simulink model "tp_thyr_rect_pm"  (R2024b)
settings: Solver=ode1be  StartTime=0.0  StopTime=simlength  FixedStep=tc  MaxStep=tc
undefined symbols (not defined in the file): CSF_11, CSF_13, CSF_5, CSF_7, Idc_traction_normalization_factor, ki_u_ctrl, kp_u_ctrl, LFu_dc, LSF_11, LSF_13, LSF_5, LSF_7, magnitude, n10, omega_grid_emulator_nom, pll_i1, pll_p, RLFu_dc, tc, Tcontrol_rect, ts, ts_ctrl_rect, ugrid_factor, Vdc_traction_normalization_factor, Vgrid_phase_normalization_factor, vn_eta_pu, vn_xi_pu, vp_xi_pu, w_grid
libraries: fl_lib x348, nesl_utility x85, ee_lib x28, single_phase_transformer_lib x6, cstblocks x3, spsEdgeDetectorLib x2
(part 1 of 8)
settings Model: SimulationMode=accelerator  Creator=dbagn  LastModifiedBy=ltnbda
settings SolverCC: NumberNewtonIterations=3  ZeroCrossControl=DisableAll  AlgebraicLoopSolver=TrustRegion  SolverResetMethod=Robust
settings DataIOCC: SaveOutput=off  SignalLogging=off  DSMLogging=off  SaveTime=off  ReturnWorkspaceOutputs=off
settings OptimizationCC: ReuseModelBlockBuffer=off  SimCompilerOptimization=on
settings DebuggingCC: UnconnectedInputMsg=warning  UnconnectedOutputMsg=warning  UnconnectedLineMsg=warning
settings ModelReferenceCC: EnableRefExpFcnMdlSchedulingChecks=on
settings SFSimCC: CustomCodeUndefinedFunction=ThrowError
settings SFSimCC: SimCustomHeaderCode=|
  | #include "math_f.h"
  | #include "mavgflt.h"
  | #include "mavgflt_simulink.h"
  | #include "bemf_obsv.h"
  | #include "bemf_obsv_simulink.h"
  | #include "bemf_obsv_load_est.h"
  | #include "bemf_obsv_load_est_simulink.h"
  | #include "dqvector_pi.h"
  | #include "dqvector_pi_simulink.h"
  | #include "sv_pwm_simulink.h"
  | #include "sv_pwm.h"
  | #include "twelve_pulse_rect.h"
  | #include "first_harmonic_tracker.h"
  | #include "first_harmonic_tracker_simulink.h"
  | #include "dqpll_thyr.h"
  | #include "dqpll_thyr_simulink.h"
  | #include "dqpll_grid.h"
  | #include "dqpll_grid_simulink.h"
  | #include "six_pulse_rect.h"
settings SFSimCC: SimUserSources=|
  | "mavgflt_simulink.c"
  | "mavgflt.c"
  | "bemf_obsv_simulink.c"
  | "bemf_obsv.c"
  | "bemf_obsv_load_est_simulink.c"
  | "bemf_obsv_load_est.c"
  | "dqvector_pi.c"
  | "dqvector_pi_simulink.c"
  | "sv_pwm_simulink.c"
  | "sv_pwm.c"
  | "twelve_pulse_rect.c"
  | "first_harmonic_tracker_simulink.c"
  | "first_harmonic_tracker.c"
  | "dqpll_thyr_simulink.c"
  | "dqpll_thyr.c"
  | "dqpll_grid_simulink.c"
  | "dqpll_grid.c"
  | "six_pulse_rect.c"
settings SFSimCC: SimUserIncludeDirs=|
  | include
  | src
settings RTWCC: GPUComputeCapability=3.5  DLArmComputeVersion=19.05

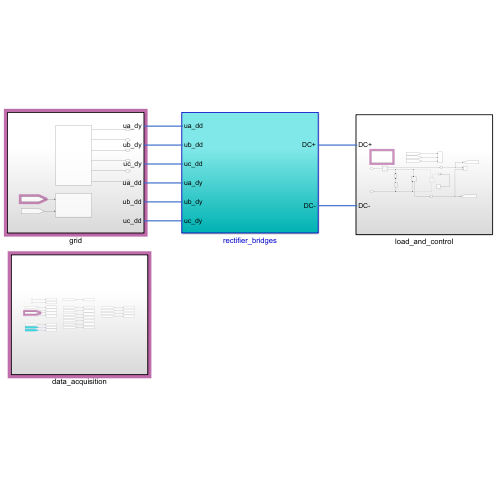
[thumbnail: Simulink's stored preview of the top-level diagram]
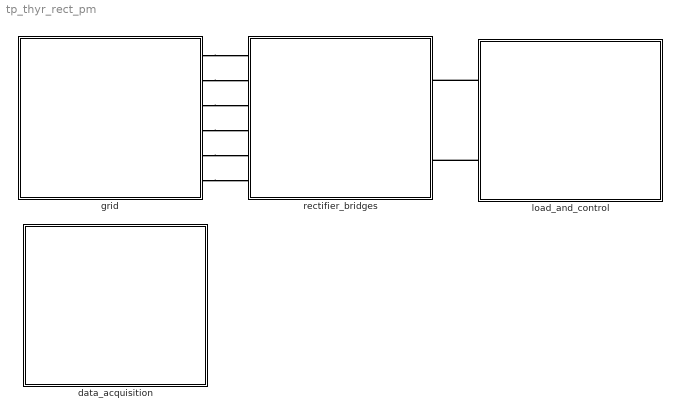
== system tp_thyr_rect_pm ==
  data_acquisition : Subsystem
  grid : Subsystem
  load_and_control : Subsystem
  rectifier_bridges : Subsystem
  connections:
  load_and_control/LConn1 -- rectifier_bridges/RConn1
  load_and_control/LConn2 -- rectifier_bridges/RConn2
  grid/RConn1 -- rectifier_bridges/LConn1
  grid/RConn2 -- rectifier_bridges/LConn2
  grid/RConn3 -- rectifier_bridges/LConn3
  grid/RConn4 -- rectifier_bridges/LConn4
  grid/RConn5 -- rectifier_bridges/LConn5
  grid/RConn6 -- rectifier_bridges/LConn6

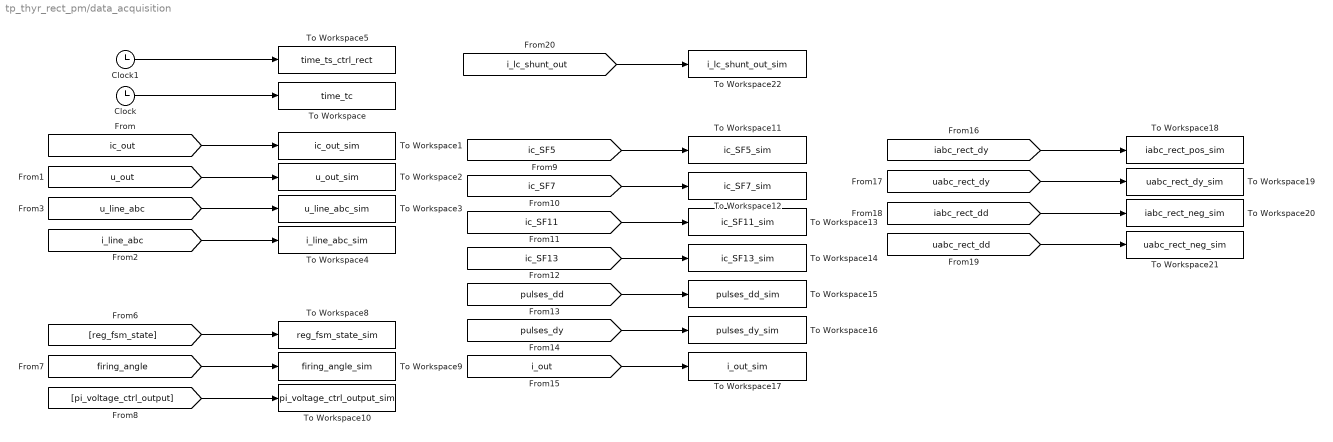
== system tp_thyr_rect_pm/data_acquisition ==
  Clock : Clock
  Clock1 : Clock
  To Workspace : ToWorkspace  VariableName=time_tc  SaveFormat=Timeseries  SampleTime=tc
      settings: MaxDataPoints=Nc
  To Workspace1 : ToWorkspace  VariableName=ic_out_sim  SaveFormat=Timeseries  SampleTime=tc
      settings: MaxDataPoints=Nc
  To Workspace10 : ToWorkspace  VariableName=pi_voltage_ctrl_output_sim  SaveFormat=Timeseries  SampleTime=ts_ctrl_rect
      settings: MaxDataPoints=Ns_ctrl_rect
  To Workspace11 : ToWorkspace  VariableName=ic_SF5_sim  SaveFormat=Timeseries  SampleTime=tc
      settings: MaxDataPoints=Nc
  To Workspace12 : ToWorkspace  VariableName=ic_SF7_sim  SaveFormat=Timeseries  SampleTime=tc
      settings: MaxDataPoints=Nc
  To Workspace13 : ToWorkspace  VariableName=ic_SF11_sim  SaveFormat=Timeseries  SampleTime=tc
      settings: MaxDataPoints=Nc
  To Workspace14 : ToWorkspace  VariableName=ic_SF13_sim  SaveFormat=Timeseries  SampleTime=tc
      settings: MaxDataPoints=Nc
  To Workspace15 : ToWorkspace  VariableName=pulses_dd_sim  SaveFormat=Timeseries  SampleTime=tc
      settings: MaxDataPoints=Nc
  To Workspace16 : ToWorkspace  VariableName=pulses_dy_sim  SaveFormat=Timeseries  SampleTime=tc
      settings: MaxDataPoints=Nc
  To Workspace17 : ToWorkspace  VariableName=i_out_sim  SaveFormat=Timeseries  SampleTime=tc
      settings: MaxDataPoints=Nc
  To Workspace18 : ToWorkspace  VariableName=iabc_rect_pos_sim  SaveFormat=Timeseries  SampleTime=tc
      settings: MaxDataPoints=Nc
  To Workspace19 : ToWorkspace  VariableName=uabc_rect_dy_sim  SaveFormat=Timeseries  SampleTime=tc
      settings: MaxDataPoints=Nc
  To Workspace2 : ToWorkspace  VariableName=u_out_sim  SaveFormat=Timeseries  SampleTime=tc
      settings: MaxDataPoints=Nc
  To Workspace20 : ToWorkspace  VariableName=iabc_rect_neg_sim  SaveFormat=Timeseries  SampleTime=tc
      settings: MaxDataPoints=Nc
  To Workspace21 : ToWorkspace  VariableName=uabc_rect_neg_sim  SaveFormat=Timeseries  SampleTime=tc
      settings: MaxDataPoints=Nc
  To Workspace22 : ToWorkspace  VariableName=i_lc_shunt_out_sim  SaveFormat=Timeseries  SampleTime=tc
      settings: MaxDataPoints=Nc
  To Workspace3 : ToWorkspace  VariableName=u_line_abc_sim  SaveFormat=Timeseries  SampleTime=tc
      settings: MaxDataPoints=Nc
  To Workspace4 : ToWorkspace  VariableName=i_line_abc_sim  SaveFormat=Timeseries  SampleTime=tc
      settings: MaxDataPoints=Nc
  To Workspace5 : ToWorkspace  VariableName=time_ts_ctrl_rect  SaveFormat=Timeseries  SampleTime=tc
      settings: MaxDataPoints=Nc
  To Workspace8 : ToWorkspace  VariableName=reg_fsm_state_sim  SaveFormat=Timeseries  SampleTime=ts_ctrl_rect
      settings: MaxDataPoints=Ns_ctrl_rect
  To Workspace9 : ToWorkspace  VariableName=firing_angle_sim  SaveFormat=Timeseries  SampleTime=ts_ctrl_rect
      settings: MaxDataPoints=Ns_ctrl_rect
  wires:
  [ic_out] -> To Workspace1/1
  Clock/1 -> To Workspace/1
  [u_line_abc] -> To Workspace3/1
  [i_line_abc] -> To Workspace4/1
  [u_out] -> To Workspace2/1
  Clock1/1 -> To Workspace5/1
  [reg_fsm_state] -> To Workspace8/1
  [firing_angle] -> To Workspace9/1
  [pi_voltage_ctrl_output] -> To Workspace10/1
  [ic_SF5] -> To Workspace11/1
  [ic_SF7] -> To Workspace12/1
  [ic_SF11] -> To Workspace13/1
  [ic_SF13] -> To Workspace14/1
  [pulses_dd] -> To Workspace15/1
  [pulses_dy] -> To Workspace16/1
  [i_out] -> To Workspace17/1
  [iabc_rect_dy] -> To Workspace18/1
  [uabc_rect_dy] -> To Workspace19/1
  [uabc_rect_dd] -> To Workspace21/1
  [iabc_rect_dd] -> To Workspace20/1
  [i_lc_shunt_out] -> To Workspace22/1

== system tp_thyr_rect_pm/grid ==
  grid_emulator : Subsystem
  instantaneus_power : Subsystem
  ua_dy : PMIOPort  Side=Right
  ub_dy : PMIOPort  Port=2  Side=Right
  uc_dy : PMIOPort  Port=3  Side=Right
  ua_dd : PMIOPort  Port=4  Side=Right
  ub_dd : PMIOPort  Port=5  Side=Right
  uc_dd : PMIOPort  Port=6  Side=Right
  wires:
  [u_line_abc] -> instantaneus_power/1(Vline)
  [i_line_abc] -> instantaneus_power/2(Iline)
  connections:
  ua_dy/RConn1 -- grid_emulator/RConn4
  ub_dy/RConn1 -- grid_emulator/RConn5
  uc_dy/RConn1 -- grid_emulator/RConn6
  ua_dd/RConn1 -- grid_emulator/RConn1
  ub_dd/RConn1 -- grid_emulator/RConn2
  uc_dd/RConn1 -- grid_emulator/RConn3

== system tp_thyr_rect_pm/load_and_control ==
  Controlled Current Source : fl_lib/Electrical/Electrical Sources/Controlled Current Source  Commented=on
  Current Sensor : fl_lib/Electrical/Electrical Sensors/Current Sensor
  Inductor : fl_lib/Electrical/Electrical Elements/Inductor  l=20e-3 H  r=0 Ohm  g=1e-9 1/Ohm  i_specify=off  i_priority=None  i=0 A  i_nominal_specify=off  i_nominal_value=1  i_nominal_unit=A  v_specify=off  v_priority=None  v=0 V  v_nominal_specify=off  v_nominal_value=1  v_nominal_unit=V  i_L_specify=off  i_L_priority=High  i_L=0 A  i_L_nominal_specify=off  i_L_nominal_value=1  i_L_nominal_unit=A
  PS-Simulink Converter : nesl_utility/PS-Simulink Converter  PhysicalDomain=network_engine_domain  SubClassName=ps_output  LeftPortType=input  RightPortType=output  PseudoPeriodic=off  Frequencies=[]  VectorFormat=1-D array  Unit=A  AffineConversion=off
  PS-Simulink Converter1 : nesl_utility/PS-Simulink Converter  PhysicalDomain=network_engine_domain  SubClassName=ps_output  LeftPortType=input  RightPortType=output  PseudoPeriodic=off  Frequencies=[]  VectorFormat=1-D array  Unit=V  AffineConversion=on
  Resistor : fl_lib/Electrical/Electrical Elements/Resistor  R=1 Ohm  i_specify=off  i_priority=None  i=0 A  i_nominal_specify=off  i_nominal_value=1  i_nominal_unit=A  v_specify=off  v_priority=None  v=0 V  v_nominal_specify=off  v_nominal_value=1  v_nominal_unit=V
  Simulink-PS Converter : nesl_utility/Simulink-PS Converter  PhysicalDomain=network_engine_domain  SubClassName=ps_input  LeftPortType=input  RightPortType=output  PseudoPeriodic=off  Frequencies=[]  NoiseDistribution=none  NoiseParameters=[]  Unit=1  AffineConversion=off  FilteringAndDerivatives=provide  SimscapeFilterOrder=1  InputFilterTimeConstant=0.001  UdotUserProvided=0
  Sine Wave : Sin  Amplitude=Idc_traction_normalization_factor/2  Bias=Idc_traction_normalization_factor/2  Frequency=pi/2  SampleTime=0
  Voltage Sensor : fl_lib/Electrical/Electrical Sensors/Voltage Sensor
  controller : Subsystem
  iu_out : Scope  NumInputPorts=2
  ui_Cout : Scope  NumInputPorts=3
  DC+ : PMIOPort  Side=Left
  DC- : PMIOPort  Port=2  Side=Left
  tag scope: i_out=global, u_out=global
  wires:
  PS-Simulink Converter/1 -> [i_out], iu_out/1  "i_out"
  PS-Simulink Converter1/1 -> [u_out], iu_out/2  "u_out"
  Sine Wave/1 -> Simulink-PS Converter/1
  [u_out] -> ui_Cout/2  "u_out"
  [ic_out] -> ui_Cout/1  "ic_out"
  [i_lc_shunt_out] -> ui_Cout/3  "i_lc_shunt_out"
  connections:
  Voltage Sensor/RConn1 -- PS-Simulink Converter1/LConn1
  Simulink-PS Converter/RConn1 -- Controlled Current Source/RConn1
  Voltage Sensor/LConn1 -- Controlled Current Source/RConn2 -- Resistor/LConn1 -- Current Sensor/RConn2
  PS-Simulink Converter/LConn1 -- Current Sensor/RConn1
  DC-/RConn1 -- Inductor/RConn1 -- Controlled Current Source/LConn1 -- Voltage Sensor/RConn2
  Inductor/LConn1 -- Resistor/RConn1
  Current Sensor/LConn1 -- DC+/RConn1

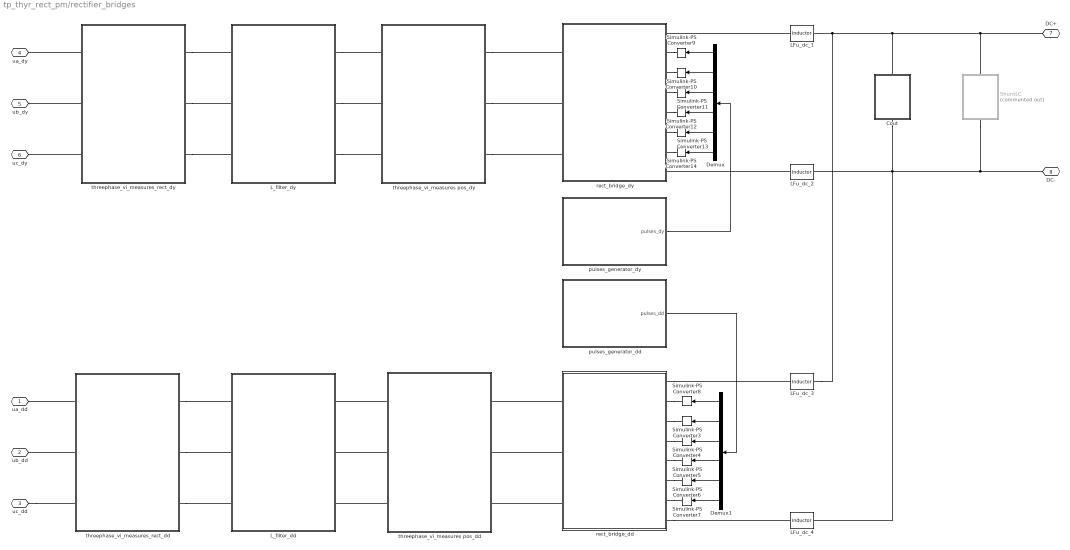
== system tp_thyr_rect_pm/rectifier_bridges ==
  Cout : Subsystem
  Demux : Demux  Outputs=6
  Demux1 : Demux  Outputs=6
  LFu_dc_{1..4} (4 alike) : fl_lib/Electrical/Electrical Elements/Inductor  l=LFu_dc/2 H  r=RLFu_dc/2 Ohm  g=1e-9 1/Ohm  i_specify=off  i_priority=None  i=0 A  i_nominal_specify=off  i_nominal_value=1  i_nominal_unit=A  v_specify=off  v_priority=None  v=0 V  v_nominal_specify=off  v_nominal_value=1  v_nominal_unit=V  i_L_specify=off  i_L_priority=High  i_L=0 A  i_L_nominal_specify=off  i_L_nominal_value=1  i_L_nominal_unit=A
  L_filter_dd : Subsystem
  L_filter_dy : Subsystem
  ShuntLC : Subsystem  Commented=on
  Simulink-PS Converter{3,5..10,12..14} (10 alike) : nesl_utility/Simulink-PS Converter  PhysicalDomain=network_engine_domain  SubClassName=ps_input  LeftPortType=input  RightPortType=output  PseudoPeriodic=off  Frequencies=[]  NoiseDistribution=none  NoiseParameters=[]  Unit=V  AffineConversion=on  FilteringAndDerivatives=provide  SimscapeFilterOrder=1  InputFilterTimeConstant=0.001  UdotUserProvided=0
  Simulink-PS Converter11 : nesl_utility/Simulink-PS Converter  PhysicalDomain=network_engine_domain  SubClassName=ps_input  LeftPortType=input  RightPortType=output  PseudoPeriodic=off  Frequencies=[]  NoiseDistribution=none  NoiseParameters=[]  Unit=V  AffineConversion=off  FilteringAndDerivatives=provide  SimscapeFilterOrder=1  InputFilterTimeConstant=0.001  UdotUserProvided=0
  Simulink-PS Converter4 : nesl_utility/Simulink-PS Converter  PhysicalDomain=network_engine_domain  SubClassName=ps_input  LeftPortType=input  RightPortType=output  PseudoPeriodic=off  Frequencies=[]  NoiseDistribution=none  NoiseParameters=[]  Unit=V  AffineConversion=off  FilteringAndDerivatives=provide  SimscapeFilterOrder=1  InputFilterTimeConstant=0.001  UdotUserProvided=0
  pulses_generator_dd : Subsystem
  pulses_generator_dy : Subsystem
  rect_bridge_dd : Subsystem
  rect_bridge_dy : Subsystem
  threephase_vi_measures pos_dd : Subsystem
  threephase_vi_measures pos_dy : Subsystem
  threephase_vi_measures_rect_dd : Subsystem
  threephase_vi_measures_rect_dy : Subsystem
  ua_dd : PMIOPort  Side=Left
  ub_dd : PMIOPort  Port=2  Side=Left
  uc_dd : PMIOPort  Port=3  Side=Left
  ua_dy : PMIOPort  Port=4  Side=Left
  ub_dy : PMIOPort  Port=5  Side=Left
  uc_dy : PMIOPort  Port=6  Side=Left
  DC+ : PMIOPort  Port=7  Side=Right
  DC- : PMIOPort  Port=8  Side=Right
  wires:
  Demux1/1 -> Simulink-PS Converter8/1
  Demux/6 -> Simulink-PS Converter14/1
  Demux1/4 -> Simulink-PS Converter5/1
  Demux1/6 -> Simulink-PS Converter7/1
  Demux1/3 -> Simulink-PS Converter4/1
  Demux/4 -> Simulink-PS Converter12/1
  Demux1/2 -> Simulink-PS Converter3/1
  Demux/1 -> Simulink-PS Converter9/1
  Demux/2 -> Simulink-PS Converter10/1
  Demux/3 -> Simulink-PS Converter11/1
  Demux1/5 -> Simulink-PS Converter6/1
  Demux/5 -> Simulink-PS Converter13/1
  pulses_generator_dd/1(pulses_dd) -> Demux1/1
  pulses_generator_dy/1(pulses_dy) -> Demux/1
  connections:
  rect_bridge_dy/LConn3 -- Simulink-PS Converter10/RConn1
  rect_bridge_dd/LConn6 -- Simulink-PS Converter6/RConn1
  rect_bridge_dd/LConn5 -- Simulink-PS Converter5/RConn1
  rect_bridge_dy/LConn5 -- Simulink-PS Converter12/RConn1
  rect_bridge_dd/LConn2 -- Simulink-PS Converter8/RConn1
  rect_bridge_dy/LConn2 -- Simulink-PS Converter9/RConn1
  rect_bridge_dd/LConn3 -- Simulink-PS Converter3/RConn1
  rect_bridge_dy/LConn4 -- Simulink-PS Converter11/RConn1
  rect_bridge_dd/LConn7 -- Simulink-PS Converter7/RConn1
  rect_bridge_dy/LConn6 -- Simulink-PS Converter13/RConn1
  rect_bridge_dy/LConn7 -- Simulink-PS Converter14/RConn1
  rect_bridge_dd/LConn4 -- Simulink-PS Converter4/RConn1
  L_filter_dy/LConn2 -- threephase_vi_measures pos_dy/LConn2
  L_filter_dy/LConn1 -- threephase_vi_measures pos_dy/LConn1
  L_filter_dy/LConn3 -- threephase_vi_measures pos_dy/LConn3
  threephase_vi_measures pos_dy/RConn1 -- rect_bridge_dy/RConn1
  threephase_vi_measures pos_dy/RConn2 -- rect_bridge_dy/RConn2
  threephase_vi_measures pos_dy/RConn3 -- rect_bridge_dy/RConn3
  rect_bridge_dd/RConn1 -- threephase_vi_measures pos_dd/RConn1
  rect_bridge_dd/RConn2 -- threephase_vi_measures pos_dd/RConn2
  rect_bridge_dd/RConn3 -- threephase_vi_measures pos_dd/RConn3
  LFu_dc_4/RConn1 -- LFu_dc_2/RConn1 -- Cout/RConn1 -- ShuntLC/RConn1 -- DC-/RConn1
  LFu_dc_1/RConn1 -- LFu_dc_3/RConn1 -- Cout/LConn1 -- ShuntLC/LConn1 -- DC+/RConn1
  LFu_dc_1/LConn1 -- rect_bridge_dy/LConn1
  LFu_dc_2/LConn1 -- rect_bridge_dy/LConn8
  rect_bridge_dd/LConn1 -- LFu_dc_3/LConn1
  rect_bridge_dd/LConn8 -- LFu_dc_4/LConn1
  threephase_vi_measures pos_dd/LConn3 -- L_filter_dd/LConn3
  threephase_vi_measures pos_dd/LConn1 -- L_filter_dd/LConn1
  threephase_vi_measures pos_dd/LConn2 -- L_filter_dd/LConn2
  threephase_vi_measures_rect_dy/RConn3 -- L_filter_dy/RConn3
  threephase_vi_measures_rect_dy/RConn2 -- L_filter_dy/RConn2
  threephase_vi_measures_rect_dy/RConn1 -- L_filter_dy/RConn1
  threephase_vi_measures_rect_dy/LConn1 -- ua_dy/RConn1
  threephase_vi_measures_rect_dy/LConn2 -- ub_dy/RConn1
  threephase_vi_measures_rect_dy/LConn3 -- uc_dy/RConn1
  threephase_vi_measures_rect_dd/LConn1 -- ua_dd/RConn1
  threephase_vi_measures_rect_dd/RConn1 -- L_filter_dd/RConn1
  threephase_vi_measures_rect_dd/RConn2 -- L_filter_dd/RConn2
  threephase_vi_measures_rect_dd/RConn3 -- L_filter_dd/RConn3
  uc_dd/RConn1 -- threephase_vi_measures_rect_dd/LConn3
  threephase_vi_measures_rect_dd/LConn2 -- ub_dd/RConn1

== system tp_thyr_rect_pm/grid/grid_emulator ==
  3ph_Dyg : Subsystem  Commented=on
  3ph_Yyg : Subsystem  Commented=on
  Controlled Voltage Source : fl_lib/Electrical/Electrical Sources/Controlled Voltage Source
  Controlled Voltage Source1 : fl_lib/Electrical/Electrical Sources/Controlled Voltage Source
  Controlled Voltage Source2 : fl_lib/Electrical/Electrical Sources/Controlled Voltage Source
  Electrical Reference : fl_lib/Electrical/Electrical Elements/Electrical Reference
  Phase Splitter : ee_lib/Connectors & References/Phase Splitter
  Phase Splitter1 : ee_lib/Connectors & References/Phase Splitter
  Phase Splitter2 : ee_lib/Connectors & References/Phase Splitter
  Simulink-PS Converter : nesl_utility/Simulink-PS Converter  PhysicalDomain=network_engine_domain  SubClassName=ps_input  LeftPortType=input  RightPortType=output  PseudoPeriodic=off  Frequencies=[]  NoiseDistribution=none  NoiseParameters=[]  Unit=V  AffineConversion=on  FilteringAndDerivatives=provide  SimscapeFilterOrder=1  InputFilterTimeConstant=0.001  UdotUserProvided=0
  Simulink-PS Converter1 : nesl_utility/Simulink-PS Converter  PhysicalDomain=network_engine_domain  SubClassName=ps_input  LeftPortType=input  RightPortType=output  PseudoPeriodic=off  Frequencies=[]  NoiseDistribution=none  NoiseParameters=[]  Unit=V  AffineConversion=on  FilteringAndDerivatives=provide  SimscapeFilterOrder=1  InputFilterTimeConstant=0.001  UdotUserProvided=0
  Simulink-PS Converter2 : nesl_utility/Simulink-PS Converter  PhysicalDomain=network_engine_domain  SubClassName=ps_input  LeftPortType=input  RightPortType=output  PseudoPeriodic=off  Frequencies=[]  NoiseDistribution=none  NoiseParameters=[]  Unit=V  AffineConversion=on  FilteringAndDerivatives=provide  SimscapeFilterOrder=1  InputFilterTimeConstant=0.001  UdotUserProvided=0
  Solver Configuration : nesl_utility/Solver Configuration  PhysicalDomain=network_engine_domain  SubClassName=solver  LeftPortType=input  RightPortType=generic  Tones=[]  Harmonics=[]  SimulateNoise=off  Profile=off  UseLocalSampling=off  EnableSwitchedLinearOptims=on  FrequencyDomain=off  UseCCode=off  RelTol=0.001  AbsTol=0.001  MinStep=1e-09  ToWorkspace=off  RevertToSquareIcSolve=off  NumHomotopyIterations=100  PhasorMode=off  PhasorModeNumHarmonics=1  ConsistencySolver=NEWTON_FTOL  IndexReductionMethod=DerivativeReplacement  DoDC=off  ResidualTolerance=1e-09  ConsistencyTolSource=GLOBAL  ConsistencyAbsTol=0.001  ConsistencyRelTol=0.001  ConsistencyTolFactor=0.001  UseLocalSolver=on  LocalSolverChoice=NE_BACKWARD_EULER_ADVANCER  ResolveIndetEquations=on  FunctionEvalNumThread=1  LocalSolverSampleTime=tc  DoFixedCost=on  MaxNonlinIter=3  MaxModeIter=2  ComputeImpulses=off  ImpulseIterations=2  LinearAlgebra=auto  LinearAlgebraNumThread=0  EquationFormulation=NE_TIME_EF  DelaysMemoryBudget=1024  AutomaticFiltering=on  FilteringTimeConstant=0.001  PartitionStorageMethod=AS_NEEDED  PartitionMemoryBudget=1024  PartitionMethod=ROBUST  MultibodyUseLocalSolver=off  MultibodyLocalSolverChoice=ODE1  MultibodyLocalSolverSampleTime=0.001
  Three-Winding Transformer (Three-Phase) : ee_lib/Passive/Transformers/Three-Winding Transformer (Three-Phase)  SRated=1.6e6 A*V  FRated=50 Hz  Winding1Connection=ee.enum.windingconnection.delta11  VRated1=400 V  Winding2Connection=ee.enum.windingconnection.delta1  VRated2=400 V  Winding3Connection=ee.enum.windingconnection.Y  VRated3=400 V  CoreType=ee.enum.coretype.threelimb  pu_Rw1=0.02  pu_Rw2=0.02  pu_Rw3=0.02  leakage_reactance_option=ee.enum.transformer_leakage.include  pu_Xl1=0.05  pu_Xl2=0.05  pu_Xl3=0.05  magnetizing_resistance_option=ee.enum.transformer_magnetizingResistance.include  pu_Rm=500  magnetizing_reactance_option=ee.enum.transformer_magnetizingReactance.include  saturation_option=ee.enum.transformer_saturation.exclude  pu_Xm=500  current_data=[0, .002, 1, 2]  magnetic_flux_data=[0, 1.2, 1.5, 1.51]  pu_X0=0.5  i1_specify=off  i1_priority=None  i1=[0, 0, 0] A  i1_nominal_specify=off  i1_nominal_value=1  i1_nominal_unit=A  i2_specify=off  i2_priority=None  i2=[0, 0, 0] A  i2_nominal_specify=off  i2_nominal_value=1  i2_nominal_unit=A  i3_specify=off  i3_priority=None  i3=[0, 0, 0] A  i3_nominal_specify=off  i3_nominal_value=1  i3_nominal_unit=A  phi_specify=off  phi_priority=None  phi=[0, 0, 0]  phi_nominal_specify=off  phi_nominal_value=1  phi_nominal_unit=1  power_dissipated_specify=off  power_dissipated_priority=None  power_dissipated=0 W  power_dissipated_nominal_specify=off  power_dissipated_nominal_value=1  power_dissipated_nominal_unit=W
      settings: InternalSimscapePortConfiguration="{\"Bottom\":[],\"Left\":[{\"id\":\"N1\",\"label\":\"~1\",\"type\":\"foundation.electrical.three_phase\"}],\"Right\":[{\"id\":\"N2\",\"label\":\"~2\",\"type\":\"foundation.electrical.three_phase\"},{\"id\":\"N3\",\"label\":\"~3\",\"type\":\"foundation.electrical.three_phase\"}],\"Top\":[]}"
  grid_emulator : Subsystem
  threephase_vi_measures : Subsystem
  ua_dd : PMIOPort  Side=Right
  ub_dd : PMIOPort  Port=2  Side=Right
  uc_dd : PMIOPort  Port=3  Side=Right
  ua_dy : PMIOPort  Port=4  Side=Right
  ub_dy : PMIOPort  Port=5  Side=Right
  uc_dy : PMIOPort  Port=6  Side=Right
  wires:
  grid_emulator/2(Vmb) -> Simulink-PS Converter1/1
  grid_emulator/3(Vmc) -> Simulink-PS Converter2/1
  grid_emulator/1(Vma) -> Simulink-PS Converter/1
  connections:
  Simulink-PS Converter/RConn1 -- Controlled Voltage Source/RConn1
  Simulink-PS Converter1/RConn1 -- Controlled Voltage Source1/RConn1
  Simulink-PS Converter2/RConn1 -- Controlled Voltage Source2/RConn1
  Electrical Reference/LConn1 -- Solver Configuration/RConn1 -- Controlled Voltage Source/RConn2 -- Controlled Voltage Source1/RConn2 -- Controlled Voltage Source2/RConn2
  Controlled Voltage Source/LConn1 -- threephase_vi_measures/LConn1
  Controlled Voltage Source1/LConn1 -- threephase_vi_measures/LConn2
  Controlled Voltage Source2/LConn1 -- threephase_vi_measures/LConn3
  Phase Splitter/RConn3 -- threephase_vi_measures/RConn1
  threephase_vi_measures/RConn2 -- Phase Splitter/RConn2
  threephase_vi_measures/RConn3 -- Phase Splitter/RConn1
  Three-Winding Transformer (Three-Phase)/LConn1 -- Phase Splitter/LConn1
  ua_dd/RConn1 -- Phase Splitter1/RConn1
  ub_dd/RConn1 -- Phase Splitter1/RConn2
  Phase Splitter1/RConn3 -- uc_dd/RConn1
  Phase Splitter2/LConn1 -- Three-Winding Transformer (Three-Phase)/RConn2
  Phase Splitter2/RConn1 -- ua_dy/RConn1
  Phase Splitter2/RConn2 -- ub_dy/RConn1
  Phase Splitter2/RConn3 -- uc_dy/RConn1
  Three-Winding Transformer (Three-Phase)/RConn1 -- Phase Splitter1/LConn1

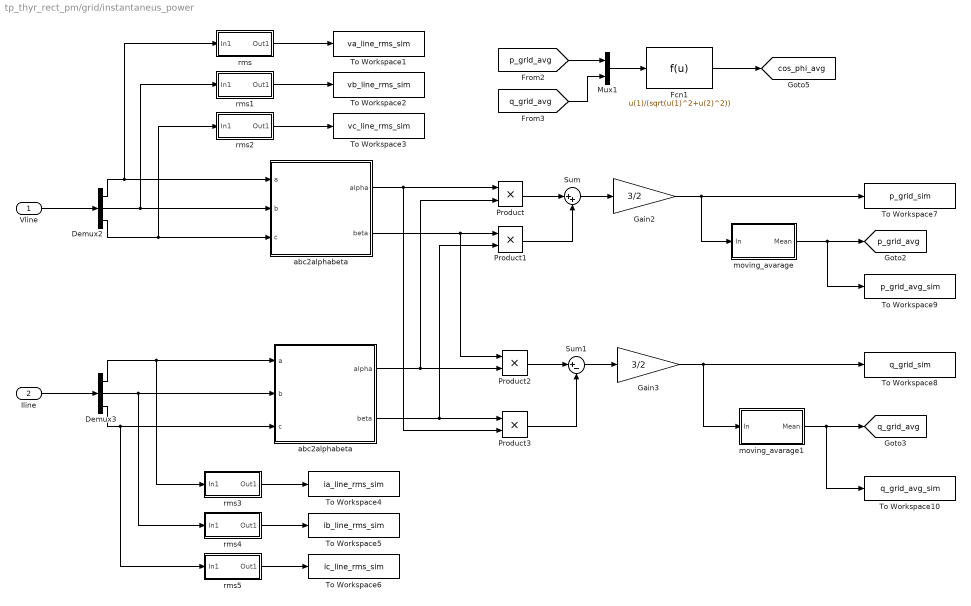
== system tp_thyr_rect_pm/grid/instantaneus_power ==
  Vline : Inport
  Iline : Inport  Port=2
  Demux2 : Demux  Outputs=3
  Demux3 : Demux  Outputs=3
  Fcn1 : Fcn  Expr=u(1)/(sqrt(u(1)^2+u(2)^2))
  Gain2 : Gain  Gain=3/2
  Gain3 : Gain  Gain=3/2
  Mux1 : Mux  Inputs=2
  Product{,1..3} (4 alike) : Product  RndMeth=Zero
  Sum : Sum  Inputs=|++
  Sum1 : Sum  Inputs=|+-
  To Workspace1 : ToWorkspace  VariableName=va_line_rms_sim  SampleTime=ts_ctrl_rect
      settings: MaxDataPoints=Ns_ctrl_rect
  To Workspace10 : ToWorkspace  VariableName=q_grid_avg_sim  SampleTime=ts_ctrl_rect
      settings: MaxDataPoints=Ns_ctrl_rect
  To Workspace2 : ToWorkspace  VariableName=vb_line_rms_sim  SampleTime=ts_ctrl_rect
      settings: MaxDataPoints=Ns_ctrl_rect
  To Workspace3 : ToWorkspace  VariableName=vc_line_rms_sim  SampleTime=ts_ctrl_rect
      settings: MaxDataPoints=Ns_ctrl_rect
  To Workspace4 : ToWorkspace  VariableName=ia_line_rms_sim  SampleTime=ts_ctrl_rect
      settings: MaxDataPoints=Ns_ctrl_rect
  To Workspace5 : ToWorkspace  VariableName=ib_line_rms_sim  SampleTime=ts_ctrl_rect
      settings: MaxDataPoints=Ns_ctrl_rect
  To Workspace6 : ToWorkspace  VariableName=ic_line_rms_sim  SampleTime=ts_ctrl_rect
      settings: MaxDataPoints=Ns_ctrl_rect
  To Workspace7 : ToWorkspace  VariableName=p_grid_sim  SampleTime=ts_ctrl_rect
      settings: MaxDataPoints=Ns_ctrl_rect
  To Workspace8 : ToWorkspace  VariableName=q_grid_sim  SampleTime=ts_ctrl_rect
      settings: MaxDataPoints=Ns_ctrl_rect
  To Workspace9 : ToWorkspace  VariableName=p_grid_avg_sim  SampleTime=ts_ctrl_rect
      settings: MaxDataPoints=Ns_ctrl_rect
  abc2alphabeta : Subsystem
  "abc2alphabeta " : Subsystem
  moving_avarage : Subsystem
  moving_avarage1 : Subsystem
  rms : Subsystem
  rms1 : Subsystem
  rms2 : Subsystem
  rms3 : Subsystem
  rms4 : Subsystem
  rms5 : Subsystem
  tag scope: cos_phi_avg=global, p_grid_avg=global, q_grid_avg=global
  wires:
  Gain3/1 -> moving_avarage1/1(In), To Workspace8/1
  Gain2/1 -> moving_avarage/1(In), To Workspace7/1
  Demux2/1 -> abc2alphabeta/1(a), rms/1(In1)
  Vline/1 -> Demux2/1
  Iline/1 -> Demux3/1
  abc2alphabeta/2("beta ") -> Product1/1, Product2/1
  "abc2alphabeta "/2("beta ") -> Product3/1, Product1/2
  abc2alphabeta/1("alpha ") -> Product/1, Product3/2
  "abc2alphabeta "/1("alpha ") -> Product2/2, Product/2
  Product/1 -> Sum/1
  Product1/1 -> Sum/2
  Product2/1 -> Sum1/1
  Product3/1 -> Sum1/2
  Sum1/1 -> Gain3/1
  Sum/1 -> Gain2/1
  Demux2/2 -> abc2alphabeta/2(b), rms1/1(In1)
  Demux2/3 -> abc2alphabeta/3(c), rms2/1(In1)
  Demux3/1 -> rms3/1(In1), "abc2alphabeta "/1(a)
  Demux3/2 -> rms4/1(In1), "abc2alphabeta "/2(b)
  Demux3/3 -> rms5/1(In1), "abc2alphabeta "/3(c)
  moving_avarage/1(Mean) -> [p_grid_avg], To Workspace9/1
  moving_avarage1/1(Mean) -> To Workspace10/1, [q_grid_avg]
  [q_grid_avg] -> Mux1/2
  Mux1/1 -> Fcn1/1
  Fcn1/1 -> [cos_phi_avg]
  [p_grid_avg] -> Mux1/1
  rms/1(Out1) -> To Workspace1/1
  rms2/1(Out1) -> To Workspace3/1
  rms1/1(Out1) -> To Workspace2/1
  rms5/1(Out1) -> To Workspace6/1
  rms4/1(Out1) -> To Workspace5/1
  rms3/1(Out1) -> To Workspace4/1

== system tp_thyr_rect_pm/load_and_control/controller ==
  Constant2 : Constant
  firing_angles : Scope
  pi_voltage_ctrl : Subsystem
  tag scope: firing_angle=global
  wires:
  [u_out] -> pi_voltage_ctrl/2(vout)
  Constant2/1 -> pi_voltage_ctrl/1(vout_ref)
  pi_voltage_ctrl/1(w) -> firing_angles/1, [firing_angle]

== system tp_thyr_rect_pm/rectifier_bridges/Cout ==
  Capacitor : fl_lib/Electrical/Electrical Elements/Capacitor  c=CFu_dc F  r=RCFu_dc Ohm  g=0 1/Ohm  i_specify=off  i_priority=None  i=0 A  i_nominal_specify=off  i_nominal_value=1  i_nominal_unit=A  v_specify=off  v_priority=None  v=0 V  v_nominal_specify=off  v_nominal_value=1  v_nominal_unit=V  vc_specify=off  vc_priority=High  vc=0 V  vc_nominal_specify=off  vc_nominal_value=1  vc_nominal_unit=V
  Current Sensor1 : fl_lib/Electrical/Electrical Sensors/Current Sensor
  PS-Simulink Converter2 : nesl_utility/PS-Simulink Converter  PhysicalDomain=network_engine_domain  SubClassName=ps_output  LeftPortType=input  RightPortType=output  PseudoPeriodic=off  Frequencies=[]  VectorFormat=1-D array  Unit=A  AffineConversion=off
  u+ : PMIOPort  Side=Left
  u- : PMIOPort  Port=2  Side=Right
  tag scope: ic_out=global
  wires:
  PS-Simulink Converter2/1 -> [ic_out]
  connections:
  Capacitor/RConn1 -- u-/RConn1
  Current Sensor1/RConn2 -- Capacitor/LConn1
  PS-Simulink Converter2/LConn1 -- Current Sensor1/RConn1
  Current Sensor1/LConn1 -- u+/RConn1

== system tp_thyr_rect_pm/rectifier_bridges/L_filter_dd ==
  Inductor : fl_lib/Electrical/Electrical Elements/Inductor  l=1e-6 H  r=0 Ohm  g=1e-9 1/Ohm  i_specify=on  i_priority=High  i=0 A  i_nominal_specify=off  i_nominal_value=1  i_nominal_unit=A  v_specify=off  v_priority=None  v=0 V  v_nominal_specify=off  v_nominal_value=1  v_nominal_unit=V  i_L_specify=off  i_L_priority=High  i_L=0 A  i_L_nominal_specify=off  i_L_nominal_value=1  i_L_nominal_unit=A
  Inductor1 : fl_lib/Electrical/Electrical Elements/Inductor  l=1e-6 H  r=0 Ohm  g=1e-9 1/Ohm  i_specify=on  i_priority=High  i=0 A  i_nominal_specify=off  i_nominal_value=1  i_nominal_unit=A  v_specify=off  v_priority=None  v=0 V  v_nominal_specify=off  v_nominal_value=1  v_nominal_unit=V  i_L_specify=off  i_L_priority=High  i_L=0 A  i_L_nominal_specify=off  i_L_nominal_value=1  i_L_nominal_unit=A
  Inductor2 : fl_lib/Electrical/Electrical Elements/Inductor  l=1e-6 H  r=0 Ohm  g=1e-9 1/Ohm  i_specify=on  i_priority=High  i=0 A  i_nominal_specify=off  i_nominal_value=1  i_nominal_unit=A  v_specify=off  v_priority=None  v=0 V  v_nominal_specify=off  v_nominal_value=1  v_nominal_unit=V  i_L_specify=off  i_L_priority=High  i_L=0 A  i_L_nominal_specify=off  i_L_nominal_value=1  i_L_nominal_unit=A
  shunt_passive_filter_11 : Subsystem  mask{CSF=CSF_11, LSF=LSF_11, RCSF=5e-3}
      mask prompts: CSF "Shunt Capacitor"; LSF "Shunt Inductor"; RCSF "Shunt Resistor"
      mask Display: disp('SPF');
  shunt_passive_filter_13 : Subsystem  mask{CSF=CSF_13, LSF=LSF_13, RCSF=5e-3}
      mask prompts: CSF "Shunt Capacitor"; LSF "Shunt Inductor"; RCSF "Shunt Resistor"
      mask Display: disp('SPF');
  shunt_passive_filter_5 : Subsystem  mask{CSF=CSF_5, LSF=LSF_5, RCSF=5e-3}
      mask prompts: CSF "Shunt Capacitor"; LSF "Shunt Inductor"; RCSF "Shunt Resistor"
      mask Display: disp('SPF');
  shunt_passive_filter_7 : Subsystem  mask{CSF=CSF_7, LSF=LSF_7, RCSF=5e-3}
      mask prompts: CSF "Shunt Capacitor"; LSF "Shunt Inductor"; RCSF "Shunt Resistor"
      mask Display: disp('SPF');
  ui_measure : Subsystem
  us_a : PMIOPort  Side=Left
  ug_a : PMIOPort  Port=2  Side=Right
  us_b : PMIOPort  Port=3  Side=Left
  ug_b : PMIOPort  Port=4  Side=Right
  us_c : PMIOPort  Port=5  Side=Left
  ug_c : PMIOPort  Port=6  Side=Right
  connections:
  ug_c/RConn1 -- ui_measure/LConn3
  ug_a/RConn1 -- ui_measure/LConn1
  ug_b/RConn1 -- ui_measure/LConn2
  Inductor2/RConn1 -- us_c/RConn1
  Inductor1/RConn1 -- us_b/RConn1
  us_a/RConn1 -- Inductor/RConn1
  shunt_passive_filter_5/RConn3 -- Inductor2/LConn1 -- shunt_passive_filter_13/RConn3 -- shunt_passive_filter_11/RConn3 -- shunt_passive_filter_7/RConn3 -- ui_measure/RConn3
  shunt_passive_filter_5/RConn2 -- Inductor1/LConn1 -- shunt_passive_filter_13/RConn2 -- shunt_passive_filter_11/RConn2 -- shunt_passive_filter_7/RConn2 -- ui_measure/RConn2
  shunt_passive_filter_5/RConn1 -- Inductor/LConn1 -- shunt_passive_filter_13/RConn1 -- shunt_passive_filter_11/RConn1 -- shunt_passive_filter_7/RConn1 -- ui_measure/RConn1

== system tp_thyr_rect_pm/rectifier_bridges/L_filter_dy ==
  Inductor : fl_lib/Electrical/Electrical Elements/Inductor  l=1e-6 H  r=0 Ohm  g=1e-9 1/Ohm  i_specify=on  i_priority=High  i=0 A  i_nominal_specify=off  i_nominal_value=1  i_nominal_unit=A  v_specify=off  v_priority=None  v=0 V  v_nominal_specify=off  v_nominal_value=1  v_nominal_unit=V  i_L_specify=off  i_L_priority=High  i_L=0 A  i_L_nominal_specify=off  i_L_nominal_value=1  i_L_nominal_unit=A
  Inductor1 : fl_lib/Electrical/Electrical Elements/Inductor  l=1e-6 H  r=0 Ohm  g=1e-9 1/Ohm  i_specify=on  i_priority=High  i=0 A  i_nominal_specify=off  i_nominal_value=1  i_nominal_unit=A  v_specify=off  v_priority=None  v=0 V  v_nominal_specify=off  v_nominal_value=1  v_nominal_unit=V  i_L_specify=off  i_L_priority=High  i_L=0 A  i_L_nominal_specify=off  i_L_nominal_value=1  i_L_nominal_unit=A
  Inductor2 : fl_lib/Electrical/Electrical Elements/Inductor  l=1e-6 H  r=0 Ohm  g=1e-9 1/Ohm  i_specify=on  i_priority=High  i=0 A  i_nominal_specify=off  i_nominal_value=1  i_nominal_unit=A  v_specify=off  v_priority=None  v=0 V  v_nominal_specify=off  v_nominal_value=1  v_nominal_unit=V  i_L_specify=off  i_L_priority=High  i_L=0 A  i_L_nominal_specify=off  i_L_nominal_value=1  i_L_nominal_unit=A
  i_SFs : Scope  NumInputPorts=4
  shunt_passive_filter_11 : Subsystem  mask{CSF=CSF_11, LSF=LSF_11, RCSF=5e-3}
      mask prompts: CSF "Shunt Capacitor"; LSF "Shunt Inductor"; RCSF "Shunt Resistor"
      mask Display: disp('SPF');
  shunt_passive_filter_13 : Subsystem  mask{CSF=CSF_13, LSF=LSF_13, RCSF=5e-3}
      mask prompts: CSF "Shunt Capacitor"; LSF "Shunt Inductor"; RCSF "Shunt Resistor"
      mask Display: disp('SPF');
  shunt_passive_filter_5 : Subsystem  mask{CSF=CSF_5, LSF=LSF_5, RCSF=5e-3}
      mask prompts: CSF "Shunt Capacitor"; LSF "Shunt Inductor"; RCSF "Shunt Resistor"
      mask Display: disp('SPF');
  shunt_passive_filter_7 : Subsystem  mask{CSF=CSF_7, LSF=LSF_7, RCSF=5e-3}
      mask prompts: CSF "Shunt Capacitor"; LSF "Shunt Inductor"; RCSF "Shunt Resistor"
      mask Display: disp('SPF');
  ui_measure : Subsystem
  us_a : PMIOPort  Side=Left
  ug_a : PMIOPort  Port=2  Side=Right
  us_b : PMIOPort  Port=3  Side=Left
  ug_b : PMIOPort  Port=4  Side=Right
  us_c : PMIOPort  Port=5  Side=Left
  ug_c : PMIOPort  Port=6  Side=Right
  wires:
  [ic_SF5] -> i_SFs/1
  [ic_SF7] -> i_SFs/2
  [ic_SF11] -> i_SFs/3
  [ic_SF13] -> i_SFs/4
  connections:
  ui_measure/RConn1 -- shunt_passive_filter_7/RConn1 -- shunt_passive_filter_11/RConn1 -- shunt_passive_filter_13/RConn1 -- Inductor/LConn1 -- shunt_passive_filter_5/RConn1
  ui_measure/RConn2 -- shunt_passive_filter_7/RConn2 -- shunt_passive_filter_11/RConn2 -- shunt_passive_filter_13/RConn2 -- Inductor1/LConn1 -- shunt_passive_filter_5/RConn2
  ui_measure/RConn3 -- shunt_passive_filter_7/RConn3 -- shunt_passive_filter_11/RConn3 -- shunt_passive_filter_13/RConn3 -- Inductor2/LConn1 -- shunt_passive_filter_5/RConn3
  us_a/RConn1 -- Inductor/RConn1
  Inductor1/RConn1 -- us_b/RConn1
  Inductor2/RConn1 -- us_c/RConn1
  ug_b/RConn1 -- ui_measure/LConn2
  ug_a/RConn1 -- ui_measure/LConn1
  ug_c/RConn1 -- ui_measure/LConn3

== system tp_thyr_rect_pm/rectifier_bridges/ShuntLC ==
  Capacitor : fl_lib/Electrical/Electrical Elements/Capacitor  c=C_shunt_dc F  r=RC_shunt_dc Ohm  g=0 1/Ohm  i_specify=off  i_priority=None  i=0 A  i_nominal_specify=off  i_nominal_value=1  i_nominal_unit=A  v_specify=off  v_priority=None  v=0 V  v_nominal_specify=off  v_nominal_value=1  v_nominal_unit=V  vc_specify=off  vc_priority=High  vc=0 V  vc_nominal_specify=off  vc_nominal_value=1  vc_nominal_unit=V
  Capacitor1 : fl_lib/Electrical/Electrical Elements/Capacitor  c=C_shunt_dc F  r=RC_shunt_dc Ohm  g=0 1/Ohm  i_specify=off  i_priority=None  i=0 A  i_nominal_specify=off  i_nominal_value=1  i_nominal_unit=A  v_specify=off  v_priority=None  v=0 V  v_nominal_specify=off  v_nominal_value=1  v_nominal_unit=V  vc_specify=off  vc_priority=High  vc=0 V  vc_nominal_specify=off  vc_nominal_value=1  vc_nominal_unit=V
  Current Sensor1 : fl_lib/Electrical/Electrical Sensors/Current Sensor
  Inductor : fl_lib/Electrical/Electrical Elements/Inductor  l=L_shunt_dc H  r=0 Ohm  g=1e-9 1/Ohm  i_specify=off  i_priority=None  i=0 A  i_nominal_specify=off  i_nominal_value=1  i_nominal_unit=A  v_specify=off  v_priority=None  v=0 V  v_nominal_specify=off  v_nominal_value=1  v_nominal_unit=V  i_L_specify=off  i_L_priority=High  i_L=0 A  i_L_nominal_specify=off  i_L_nominal_value=1  i_L_nominal_unit=A
  PS-Simulink Converter2 : nesl_utility/PS-Simulink Converter  PhysicalDomain=network_engine_domain  SubClassName=ps_output  LeftPortType=input  RightPortType=output  PseudoPeriodic=off  Frequencies=[]  VectorFormat=1-D array  Unit=A  AffineConversion=off
  u+ : PMIOPort  Side=Left
  u- : PMIOPort  Port=2  Side=Right
  tag scope: i_lc_shunt_out=global
  wires:
  PS-Simulink Converter2/1 -> [i_lc_shunt_out]
  connections:
  Current Sensor1/LConn1 -- u+/RConn1
  PS-Simulink Converter2/LConn1 -- Current Sensor1/RConn1
  Current Sensor1/RConn2 -- Capacitor1/LConn1 -- Capacitor/LConn1
  Capacitor/RConn1 -- Capacitor1/RConn1 -- Inductor/LConn1
  Inductor/RConn1 -- u-/RConn1

== system tp_thyr_rect_pm/rectifier_bridges/pulses_generator_dd ==
  C-caller ctrl : Subsystem
  Step : Step  Time=0  Before=1  After=0
  pll : Subsystem
  pulses_dd : Outport
  wires:
  [firing_angle] -> C-caller ctrl/1(alpha)
  C-caller ctrl/1(pulses_dy) -> pulses_dd/1
  Step/1 -> C-caller ctrl/3(Block)
  pll/1(grid_phase_hat) -> C-caller ctrl/2(grid_phase)

== system tp_thyr_rect_pm/rectifier_bridges/pulses_generator_dy ==
  C-caller ctrl : Subsystem
  Step : Step  Time=0  Before=1  After=0
  pll : Subsystem
  pulses_dy : Outport
  wires:
  pll/1(grid_phase_hat) -> C-caller ctrl/2(grid_phase)
  Step/1 -> C-caller ctrl/3(Block)
  C-caller ctrl/1(pulses_dy) -> pulses_dy/1
  [firing_angle] -> C-caller ctrl/1(alpha)

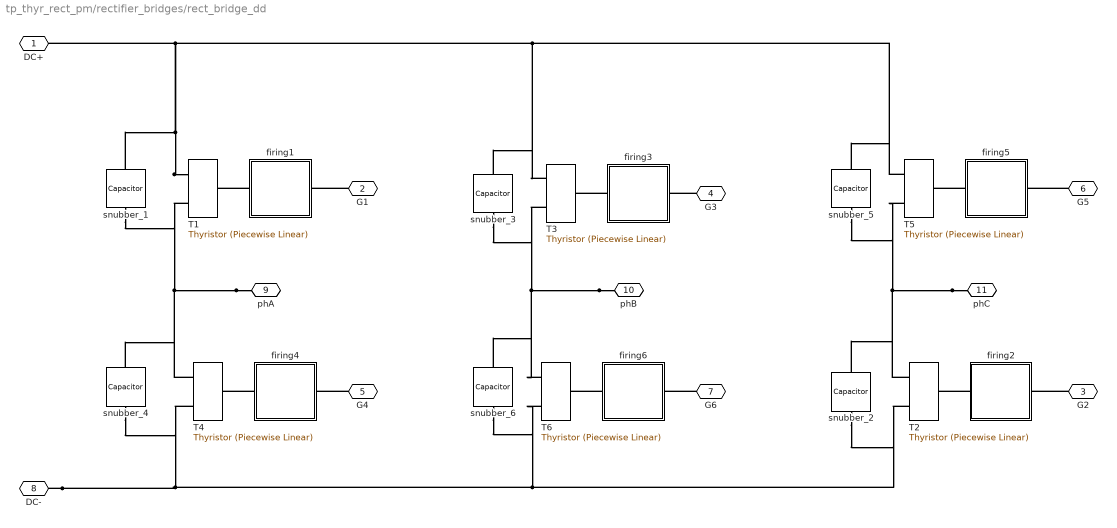
== system tp_thyr_rect_pm/rectifier_bridges/rect_bridge_dd ==
  T{1..6} (6 alike) : ee_lib/Semiconductors & Converters/Thyristor (Piecewise Linear)  port_option=ee.enum.controlport.ps  Vf=0.8 V  Ron=0.001 Ohm  Goff=1e-5 1/Ohm  Vgt=6 V  Ih=1 A  diode_param=1  diode_Vf=0.8 V  diode_Ron=0.001 Ohm  diode_Goff=1e-5 1/Ohm  diode_C=50e-9 F  diode_iRM=-235 A  diode_iF=300 A  diode_idot=-50 A/us  diode_trr_param=1  diode_trr_factor=3  diode_trr=15 us  diode_Qrr=1500 s*uA  iak_specify=off  iak_priority=None  iak=0 A  iak_nominal_specify=off  iak_nominal_value=1  iak_nominal_unit=A  vak_specify=off  vak_priority=None  vak=0 V  vak_nominal_specify=off  vak_nominal_value=1  vak_nominal_unit=V  vgk_specify=off  vgk_priority=None  vgk=0 V  vgk_nominal_specify=off  vgk_nominal_value=1  vgk_nominal_unit=V  thermal_loss_option=2  Von_data=[0, 1.1, 1.3, 1.45, 1.75, 2.25, 2.7; 0, 1, 1.15, 1.35, 1.7, 2.35, 3] V  Tj=[298.15, 398.15] K  Iout_data=[0, 10, 50, 100, 200, 400, 600] A  Eon_data=[0, .29, 1.43, 2.86, 5.71, 13.14, 22.86; 0, .57, 2.63, 5.14, 10.29, 20.57, 30.29] * 1e-3 J  Tj_loss=[298.15, 398.15] K  Iout_data_loss=[0, .1, 1, 5, 10, 20, 40, 70, 100] A  Eon_scalar=22.86e-3 J  Eoff_natural_commutation=10e-3 J  Voff=300 V  Iout_scalar=600 A  onCurrentMeasDelay=1e-4 s  diodeModelType=ee.enum.converters.diodeModelType.pwl  diodeTableType=ee.enum.diode.tableType.IfMat  diode_IfMat=[.07, .12, .19, 1.75, 4.24, 7.32, 11.2; .16, .3, .72, 2.14, 4.02, 6.35, 9.12] A  diode_VfMat=[.9, 1.15, 1.25, 1.5, 1.75, 2.17, 2.6, 2.85; .58, .68, .75, 1.1, 1.38, 1.77, 2.27, 2.7] V  diode_TjVec=[25, 125] degC  diode_VfVec=[.5, .7, .9, 1.3, 1.7, 2.1, 2.5] V  diode_IfVec=[.1, .2, .5, 1, 2, 4, 7, 10] A  diode_rec_loss_model=ee.enum.diode.reverseRecoveryModel.fixed  diode_ErecVal=0 J  diode_scaleWithIandV=true  diode_ErecMat=zeros(2, 3) J  diode_TjrecVec=[298.15, 398.15] K  diode_IfrecVec=[.1, 1, 10] A  diode_IrecVal=10 A  diode_VrecVal=10 V  diode_tFilter=1 / 1000 / 100 s  thermal_network_parameterization=ee.enum.thermalNetworkTopology.external  Rth=[.08, .5] K/W  Rth_Cauer=[.08, .1, .5] K/W  Rth_Foster=[.08, .14, .22, .16] K/W  thermal_mass_parameterization=ee.enum.thermalNetwork.timeconstant  thermal_mass=[.01, .5] J/K  thermal_mass_Cauer=[.01, .1, .5] J/K  thermal_mass_Foster=[.001, .005, .05, .5] J/K  thermal_time_constant=[.001, .2] s  thermal_time_constant_Cauer=[.001, .1, .2] s  thermal_time_constant_Foster=[7e-05, .0007, .01, .08] s  thermal_mass_initial_temperatures=[25, 25] degC  thermal_mass_initial_temperatures_Cauer=[25, 25, 25] degC  junction_thermal_mass=0.01 J/K  Tvec_initial_Foster=[25, 25, 25, 25] degC  junction_temperature_specify=off  junction_temperature_priority=None  junction_temperature=25 degC  junction_temperature_nominal_specify=off  junction_temperature_nominal_value=1  junction_temperature_nominal_unit=degC  Qj_specify=off  Qj_priority=None  Qj=0 W  Qj_nominal_specify=off  Qj_nominal_value=1  Qj_nominal_unit=W  accumulatedSwitchingLosses_specify=off  accumulatedSwitchingLosses_priority=None  accumulatedSwitchingLosses=0 J
      settings: InternalSimscapePortConfiguration="{\"Bottom\":[],\"Left\":[{\"id\":\"G\",\"label\":\"\",\"type\":\"input\"}],\"Right\":[{\"id\":\"A\",\"label\":\"\",\"type\":\"foundation.electrical.electrical\"},{\"id\":\"K\",\"label\":\"\",\"type\":\"foundation.electrical.electrical\"}],\"Top\":[]}"
  firing1 : Subsystem
  firing2 : Subsystem
  firing3 : Subsystem
  firing4 : Subsystem
  firing5 : Subsystem
  firing6 : Subsystem
  snubber_{1..6} (6 alike) : fl_lib/Electrical/Electrical Elements/Capacitor  c=Csnubber_scr F  r=Rsnubber_scr Ohm  g=0 1/Ohm  i_specify=off  i_priority=None  i=0 A  i_nominal_specify=off  i_nominal_value=1  i_nominal_unit=A  v_specify=off  v_priority=None  v=0 V  v_nominal_specify=off  v_nominal_value=1  v_nominal_unit=V  vc_specify=off  vc_priority=High  vc=0 V  vc_nominal_specify=off  vc_nominal_value=1  vc_nominal_unit=V
  DC+ : PMIOPort  Side=Left
  G1 : PMIOPort  Port=2  Side=Left
  G2 : PMIOPort  Port=3  Side=Left
  G3 : PMIOPort  Port=4  Side=Left
  G4 : PMIOPort  Port=5  Side=Left
  G5 : PMIOPort  Port=6  Side=Left
  G6 : PMIOPort  Port=7  Side=Left
  DC- : PMIOPort  Port=8  Side=Left
  phA : PMIOPort  Port=9  Side=Right
  phB : PMIOPort  Port=10  Side=Right
  phC : PMIOPort  Port=11  Side=Right
  connections:
  firing6/RConn1 -- T6/LConn1
  firing5/RConn1 -- T5/LConn1
  firing4/RConn1 -- T4/LConn1
  firing3/RConn1 -- T3/LConn1
  firing2/RConn1 -- T2/LConn1
  firing1/RConn1 -- T1/LConn1
  G6/RConn1 -- firing6/LConn1
  G5/RConn1 -- firing5/LConn1
  G4/RConn1 -- firing4/LConn1
  G3/RConn1 -- firing3/LConn1
  G2/RConn1 -- firing2/LConn1
  G1/RConn1 -- firing1/LConn1
  DC-/RConn1 -- T4/RConn1 -- snubber_4/RConn1 -- T6/RConn1 -- snubber_6/RConn1 -- snubber_2/RConn1 -- T2/RConn1
  phB/RConn1 -- T6/RConn2 -- snubber_6/LConn1 -- snubber_3/RConn1 -- T3/RConn1
  phC/RConn1 -- T5/RConn1 -- snubber_5/RConn1 -- snubber_2/LConn1 -- T2/RConn2
  phA/RConn1 -- T4/RConn2 -- snubber_4/LConn1 -- snubber_1/RConn1 -- T1/RConn1
  T1/RConn2 -- snubber_1/LConn1 -- T3/RConn2 -- snubber_3/LConn1 -- T5/RConn2 -- snubber_5/LConn1 -- DC+/RConn1

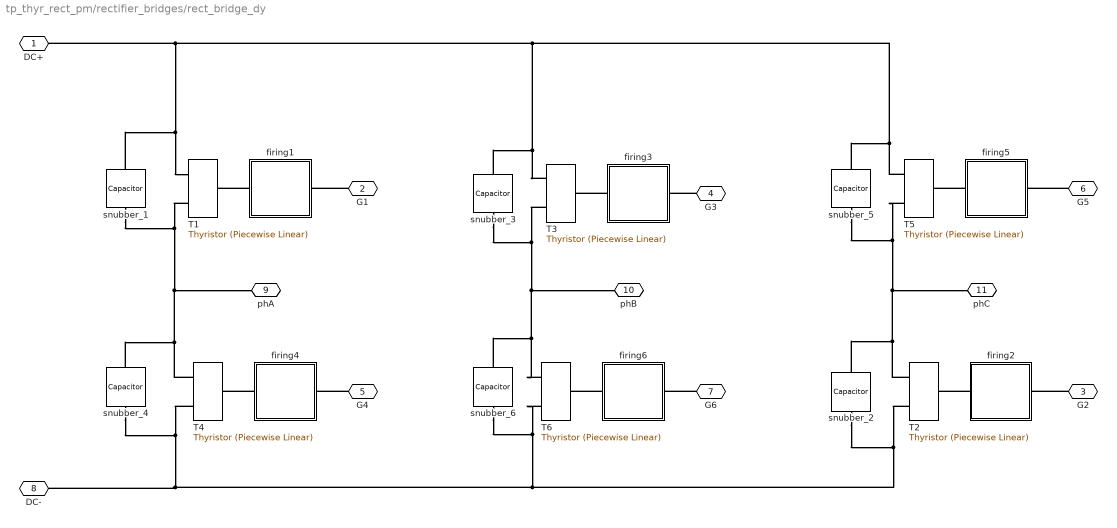
== system tp_thyr_rect_pm/rectifier_bridges/rect_bridge_dy ==
  T{1..6} (6 alike) : ee_lib/Semiconductors & Converters/Thyristor (Piecewise Linear)  port_option=ee.enum.controlport.ps  Vf=0.8 V  Ron=0.001 Ohm  Goff=1e-5 1/Ohm  Vgt=6 V  Ih=1 A  diode_param=1  diode_Vf=0.8 V  diode_Ron=0.001 Ohm  diode_Goff=1e-5 1/Ohm  diode_C=50e-9 F  diode_iRM=-235 A  diode_iF=300 A  diode_idot=-50 A/us  diode_trr_param=1  diode_trr_factor=3  diode_trr=15 us  diode_Qrr=1500 s*uA  iak_specify=off  iak_priority=None  iak=0 A  iak_nominal_specify=off  iak_nominal_value=1  iak_nominal_unit=A  vak_specify=off  vak_priority=None  vak=0 V  vak_nominal_specify=off  vak_nominal_value=1  vak_nominal_unit=V  vgk_specify=off  vgk_priority=None  vgk=0 V  vgk_nominal_specify=off  vgk_nominal_value=1  vgk_nominal_unit=V  thermal_loss_option=2  Von_data=[0, 1.1, 1.3, 1.45, 1.75, 2.25, 2.7; 0, 1, 1.15, 1.35, 1.7, 2.35, 3] V  Tj=[298.15, 398.15] K  Iout_data=[0, 10, 50, 100, 200, 400, 600] A  Eon_data=[0, .29, 1.43, 2.86, 5.71, 13.14, 22.86; 0, .57, 2.63, 5.14, 10.29, 20.57, 30.29] * 1e-3 J  Tj_loss=[298.15, 398.15] K  Iout_data_loss=[0, .1, 1, 5, 10, 20, 40, 70, 100] A  Eon_scalar=22.86e-3 J  Eoff_natural_commutation=10e-3 J  Voff=300 V  Iout_scalar=600 A  onCurrentMeasDelay=1e-4 s  diodeModelType=ee.enum.converters.diodeModelType.pwl  diodeTableType=ee.enum.diode.tableType.IfMat  diode_IfMat=[.07, .12, .19, 1.75, 4.24, 7.32, 11.2; .16, .3, .72, 2.14, 4.02, 6.35, 9.12] A  diode_VfMat=[.9, 1.15, 1.25, 1.5, 1.75, 2.17, 2.6, 2.85; .58, .68, .75, 1.1, 1.38, 1.77, 2.27, 2.7] V  diode_TjVec=[25, 125] degC  diode_VfVec=[.5, .7, .9, 1.3, 1.7, 2.1, 2.5] V  diode_IfVec=[.1, .2, .5, 1, 2, 4, 7, 10] A  diode_rec_loss_model=ee.enum.diode.reverseRecoveryModel.fixed  diode_ErecVal=0 J  diode_scaleWithIandV=true  diode_ErecMat=zeros(2, 3) J  diode_TjrecVec=[298.15, 398.15] K  diode_IfrecVec=[.1, 1, 10] A  diode_IrecVal=10 A  diode_VrecVal=10 V  diode_tFilter=1 / 1000 / 100 s  thermal_network_parameterization=ee.enum.thermalNetworkTopology.external  Rth=[.08, .5] K/W  Rth_Cauer=[.08, .1, .5] K/W  Rth_Foster=[.08, .14, .22, .16] K/W  thermal_mass_parameterization=ee.enum.thermalNetwork.timeconstant  thermal_mass=[.01, .5] J/K  thermal_mass_Cauer=[.01, .1, .5] J/K  thermal_mass_Foster=[.001, .005, .05, .5] J/K  thermal_time_constant=[.001, .2] s  thermal_time_constant_Cauer=[.001, .1, .2] s  thermal_time_constant_Foster=[7e-05, .0007, .01, .08] s  thermal_mass_initial_temperatures=[25, 25] degC  thermal_mass_initial_temperatures_Cauer=[25, 25, 25] degC  junction_thermal_mass=0.01 J/K  Tvec_initial_Foster=[25, 25, 25, 25] degC  junction_temperature_specify=off  junction_temperature_priority=None  junction_temperature=25 degC  junction_temperature_nominal_specify=off  junction_temperature_nominal_value=1  junction_temperature_nominal_unit=degC  Qj_specify=off  Qj_priority=None  Qj=0 W  Qj_nominal_specify=off  Qj_nominal_value=1  Qj_nominal_unit=W  accumulatedSwitchingLosses_specify=off  accumulatedSwitchingLosses_priority=None  accumulatedSwitchingLosses=0 J
      settings: InternalSimscapePortConfiguration="{\"Bottom\":[],\"Left\":[{\"id\":\"G\",\"label\":\"\",\"type\":\"input\"}],\"Right\":[{\"id\":\"A\",\"label\":\"\",\"type\":\"foundation.electrical.electrical\"},{\"id\":\"K\",\"label\":\"\",\"type\":\"foundation.electrical.electrical\"}],\"Top\":[]}"
  firing1 : Subsystem
  firing2 : Subsystem
  firing3 : Subsystem
  firing4 : Subsystem
  firing5 : Subsystem
  firing6 : Subsystem
  snubber_{1..6} (6 alike) : fl_lib/Electrical/Electrical Elements/Capacitor  c=Csnubber_scr F  r=Rsnubber_scr Ohm  g=0 1/Ohm  i_specify=off  i_priority=None  i=0 A  i_nominal_specify=off  i_nominal_value=1  i_nominal_unit=A  v_specify=off  v_priority=None  v=0 V  v_nominal_specify=off  v_nominal_value=1  v_nominal_unit=V  vc_specify=off  vc_priority=High  vc=0 V  vc_nominal_specify=off  vc_nominal_value=1  vc_nominal_unit=V
  DC+ : PMIOPort  Side=Left
  G1 : PMIOPort  Port=2  Side=Left
  G2 : PMIOPort  Port=3  Side=Left
  G3 : PMIOPort  Port=4  Side=Left
  G4 : PMIOPort  Port=5  Side=Left
  G5 : PMIOPort  Port=6  Side=Left
  G6 : PMIOPort  Port=7  Side=Left
  DC- : PMIOPort  Port=8  Side=Left
  phA : PMIOPort  Port=9  Side=Right
  phB : PMIOPort  Port=10  Side=Right
  phC : PMIOPort  Port=11  Side=Right
  connections:
  DC+/RConn1 -- snubber_5/LConn1 -- T5/RConn2 -- snubber_3/LConn1 -- T3/RConn2 -- snubber_1/LConn1 -- T1/RConn2
  T1/RConn1 -- snubber_1/RConn1 -- snubber_4/LConn1 -- T4/RConn2 -- phA/RConn1
  T2/RConn2 -- snubber_2/LConn1 -- snubber_5/RConn1 -- T5/RConn1 -- phC/RConn1
  T3/RConn1 -- snubber_3/RConn1 -- snubber_6/LConn1 -- T6/RConn2 -- phB/RConn1
  T2/RConn1 -- snubber_2/RConn1 -- snubber_6/RConn1 -- T6/RConn1 -- snubber_4/RConn1 -- T4/RConn1 -- DC-/RConn1
  G1/RConn1 -- firing1/LConn1
  G2/RConn1 -- firing2/LConn1
  G3/RConn1 -- firing3/LConn1
  G4/RConn1 -- firing4/LConn1
  G5/RConn1 -- firing5/LConn1
  G6/RConn1 -- firing6/LConn1
  firing1/RConn1 -- T1/LConn1
  firing2/RConn1 -- T2/LConn1
  firing3/RConn1 -- T3/LConn1
  firing4/RConn1 -- T4/LConn1
  firing5/RConn1 -- T5/LConn1
  firing6/RConn1 -- T6/LConn1
